simulink library "CustomLibrary"  (R2018b)
settings: Solver=ode45  StartTime=0.0  StopTime=10.0  RelTol=1e-3  EnableMultiTasking=on
libraries: simulink x1, CustomLib x1
settings Model: Creator=Rose  LastModifiedBy=Rose
settings DataIOCC: LimitDataPoints=on  SaveFormat=Array  SignalLoggingSaveFormat=ModelDataLogs
settings OptimizationCC: ExpressionDepthLimit=2147483647  LifeSpan=inf
settings DebuggingCC: UnderspecifiedInitializationDetection=Classic  MergeDetectMultiDrivingBlocksExec=none  SolverPrmCheckMsg=warning  FcnCallInpInsideContextMsg=warning  AllowSymbolicDim=off  StateNameClashWarn=warning  LibraryContextMissingDiagnostic=none  SFUnexpectedBacktrackingDiag=warning  SFNoUnconditionalDefaultTransitionDiag=warning  SFExecutionAtInitializationDiag=none
settings HardwareCC: ProdBitPerPointer=32  ProdBitPerSizeT=32  ProdBitPerPtrDiffT=32  ProdLargestAtomicFloat=None  ProdIntDivRoundTo=Undefined  ProdEndianess=Unspecified  ProdWordSize=32  ProdHWDeviceType=32-bit Generic
settings ModelReferenceCC: PropagateSignalLabelsOutOfModel=off
settings SFSimCC: SimUseLocalCustomCode=off
settings RTWCC: RTWUseLocalCustomCode=off
settings CodeAppCC: StateflowObjectComments=on
settings GRTTargetCC: TargetLangStandard=C89/C90 (ANSI)  GeneratePreprocessorConditionals=Disable all  CombineOutputUpdateFcns=off  GRTInterface=on
settings ConfigComp: CovMetricSettings=dw  CovHtmlReporting=on  CovSaveCumulativeToWorkspaceVar=on  CovSaveSingleToWorkspaceVar=on  CovExternalEMLEnable=off

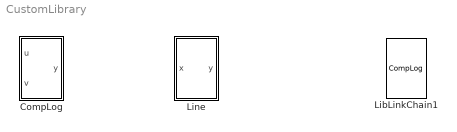
== system CustomLibrary ==
  CompLog : Subsystem
  LibLinkChain1 : CustomLib/MaskedSubsystems/CompLog  SystemSampleTime=-1
  Line : Subsystem  mask(Line){m=2, b=-1}
      mask prompts: m "Slope:"; b "Intercept:"
      mask help:
      | Models the equation for a line, y = mx + b.
      | The slope and intercept are mask block parameters.
      mask Help:
      | Enter the slope (m) and intercept (b) in the
      | block dialog parameter fields.
      | 
      | The block generates y for a given input x.
      mask Display: plot([0 1],[0 m]+(m<0))

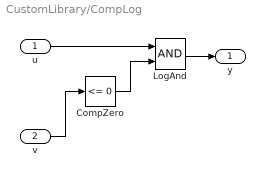
== system CustomLibrary/CompLog ==
  u : Inport  OutDataTypeStr=boolean
  v : Inport  Port=2  OutDataTypeStr=double
  CompZero : simulink/Logic and Bit Operations/Compare To Zero  relop=<=  OutDataTypeStr=uint8
  LogAnd : Logic  AllPortsSameDT=off  OutDataTypeStr=boolean
  y : Outport  OutDataTypeStr=boolean
  wires:
  LogAnd/1 -> y/1
  u/1 -> LogAnd/1
  v/1 -> CompZero/1
  CompZero/1 -> LogAnd/2

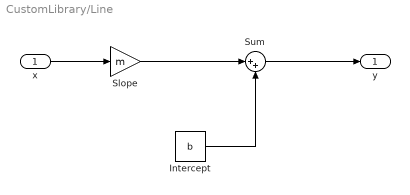
== system CustomLibrary/Line ==
  x : Inport
  Intercept : Constant  Value=b
  Slope : Gain  Gain=m
  Sum : Sum  Inputs=|++
  y : Outport
  wires:
  Intercept/1 -> Sum/2
  x/1 -> Slope/1
  Slope/1 -> Sum/1
  Sum/1 -> y/1
